simulink model "LR_RL"  (R2021a)
settings: Solver=FixedStepAuto  StartTime=0.0  StopTime=T  FixedStep=Ts  RelTol=1e-3
undefined symbols (not defined in the file): isTerminate, max_theta_error, max_x_error, max_y_error, pLander, references, u0, xpos0
libraries: simulink x8, rllib x1
settings Model: SimulationMode=accelerator  Creator=The MathWorks, Inc.  LastModifiedBy=ldy
settings DataIOCC: ReturnWorkspaceOutputs=off

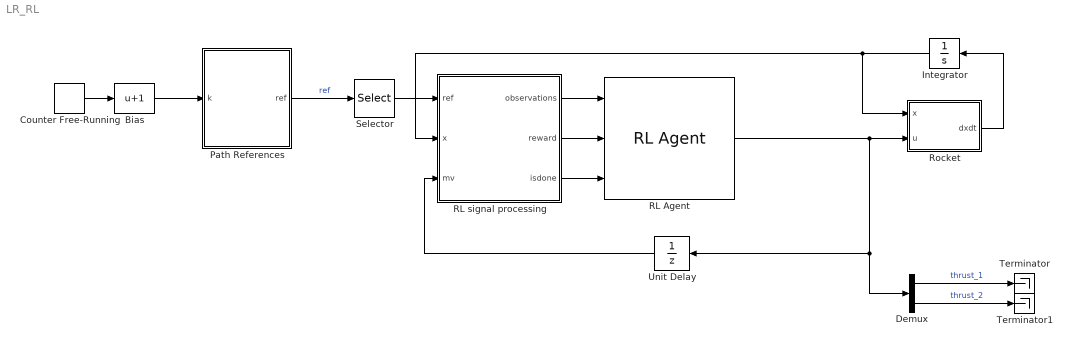
== system LR_RL ==
  Bias : Bias  Bias=1
  Counter Free-Running : simulink/Sources/Counter Free-Running  NumBits=16  tsamp=Ts
  Demux : Demux  Outputs=2
  Integrator : Integrator  InitialCondition=[xpos0;60;0;0;0;0]
  Path References : MATLAB Function  TreatAsAtomicUnit=on
  RL Agent : rllib/RL Agent  Agent=agent  ExternalActionAsInput=off  ProvideCumRwd=off  TreatAsDirectFeedthrough=on
  RL signal processing : Subsystem
  Rocket : MATLAB Function  TreatAsAtomicUnit=on
  Selector : Selector  InputPortWidth=66  IndexOptions=Index vector (dialog)  Indices=[1 2 3 4 5 6]  OutputSizes=1
  Terminator : Terminator
  Terminator1 : Terminator
  Unit Delay : UnitDelay  InitialCondition=u0  SampleTime=-1  HasFrameUpgradeWarning=on
  wires:
  Rocket/1(dxdt) -> Integrator/1
  Integrator/1 -> RL signal processing/2(x), Rocket/1(x)
  Path References/1(ref) -> Selector/1  "ref"
  Counter Free-Running/1 -> Bias/1
  Bias/1 -> Path References/1(k)
  RL signal processing/1(observations) -> RL Agent/1
  RL signal processing/3(isdone) -> RL Agent/3
  RL signal processing/2(reward) -> RL Agent/2
  Selector/1 -> RL signal processing/1(ref)
  Unit Delay/1 -> RL signal processing/3(mv)
  RL Agent/1 -> Unit Delay/1, Demux/1, Rocket/2(u)
  Demux/1 -> Terminator/1  "thrust_1"
  Demux/2 -> Terminator1/1  "thrust_2"

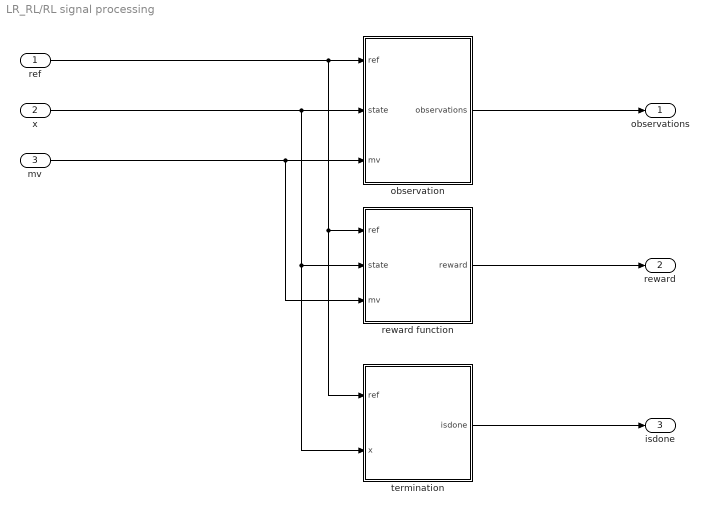
== system LR_RL/RL signal processing ==
  ref : Inport
  x : Inport  Port=2
  mv : Inport  Port=3
  observation : Subsystem
  reward function : Subsystem
  termination : Subsystem
  observations : Outport
  reward : Outport  Port=2
  isdone : Outport  Port=3
  wires:
  observation/1(observations) -> observations/1
  termination/1(isdone) -> isdone/1
  reward function/1(reward) -> reward/1
  ref/1 -> termination/1(ref), reward function/1(ref), observation/1(ref)
  x/1 -> termination/2(x), reward function/2(state), observation/2(state)
  mv/1 -> reward function/3(mv), observation/3(mv)

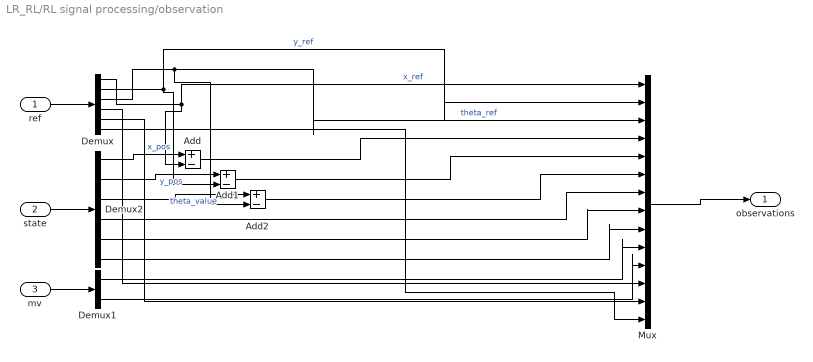
== system LR_RL/RL signal processing/observation ==
  ref : Inport
  state : Inport  Port=2
  mv : Inport  Port=3
  Add : Sum  Inputs=+-
  Add1 : Sum  Inputs=+-
  Add2 : Sum  Inputs=+-
  Demux : Demux  Outputs=6
  Demux1 : Demux  Outputs=2
  Demux2 : Demux  Outputs=6
  Mux : Mux  Inputs=14
  observations : Outport
  wires:
  ref/1 -> Demux/1
  Mux/1 -> observations/1
  mv/1 -> Demux1/1
  state/1 -> Demux2/1
  Demux/1 -> Add/2, Mux/1  "x_ref"
  Demux/2 -> Mux/2, Add1/2  "y_ref"
  Demux/3 -> Add2/2, Mux/3  "theta_ref"
  Demux2/4 -> Mux/7
  Demux2/5 -> Mux/8
  Demux2/6 -> Mux/9
  Demux1/1 -> Mux/10
  Demux1/2 -> Mux/11
  Demux2/1 -> Add/1  "x_pos"
  Add/1 -> Mux/4
  Demux2/2 -> Add1/1  "y_pos"
  Add1/1 -> Mux/5
  Demux2/3 -> Add2/1  "theta_value"
  Add2/1 -> Mux/6
  Demux/4 -> Mux/12
  Demux/5 -> Mux/13
  Demux/6 -> Mux/14

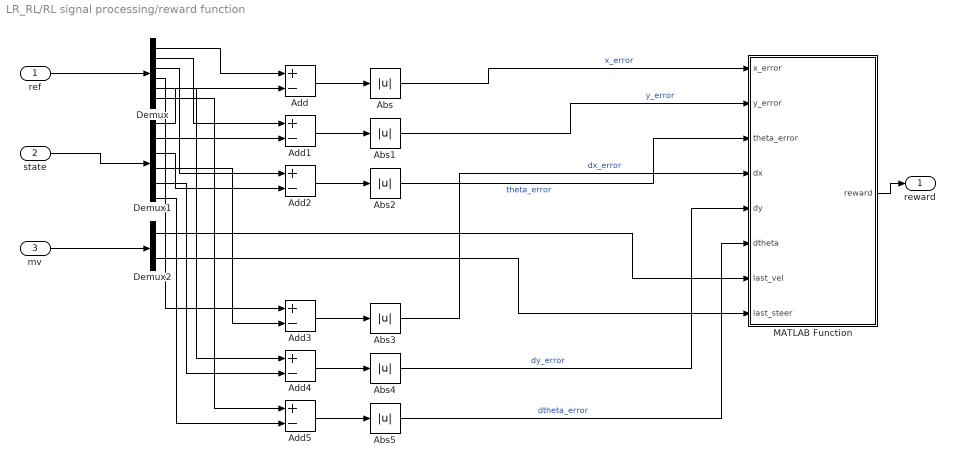
== system LR_RL/RL signal processing/reward function ==
  ref : Inport
  state : Inport  Port=2
  mv : Inport  Port=3
  Abs{,1..5} (6 alike) : Abs
  Add{,1..5} (6 alike) : Sum  Inputs=+-
  Demux : Demux  Outputs=6
  Demux1 : Demux  Outputs=6
  Demux2 : Demux  Outputs=2
  MATLAB Function : MATLAB Function  TreatAsAtomicUnit=on
  reward : Outport
  wires:
  MATLAB Function/1(reward) -> reward/1
  ref/1 -> Demux/1
  state/1 -> Demux1/1
  Demux/1 -> Add/1
  Demux/2 -> Add1/1
  Demux/3 -> Add2/1
  Demux1/1 -> Add/2
  Demux1/2 -> Add1/2
  Demux1/3 -> Add2/2
  Add/1 -> Abs/1
  Add1/1 -> Abs1/1
  Add2/1 -> Abs2/1
  mv/1 -> Demux2/1
  Abs/1 -> MATLAB Function/1(x_error)  "x_error"
  Abs1/1 -> MATLAB Function/2(y_error)  "y_error"
  Abs2/1 -> MATLAB Function/3(theta_error)  "theta_error"
  Demux2/1 -> MATLAB Function/7(last_vel)
  Demux2/2 -> MATLAB Function/8(last_steer)
  Add3/1 -> Abs3/1
  Add4/1 -> Abs4/1
  Add5/1 -> Abs5/1
  Demux/4 -> Add3/1
  Demux1/4 -> Add3/2
  Demux/5 -> Add4/1
  Demux1/5 -> Add4/2
  Demux/6 -> Add5/1
  Demux1/6 -> Add5/2
  Abs3/1 -> MATLAB Function/4(dx)  "dx_error"
  Abs4/1 -> MATLAB Function/5(dy)  "dy_error"
  Abs5/1 -> MATLAB Function/6(dtheta)  "dtheta_error"

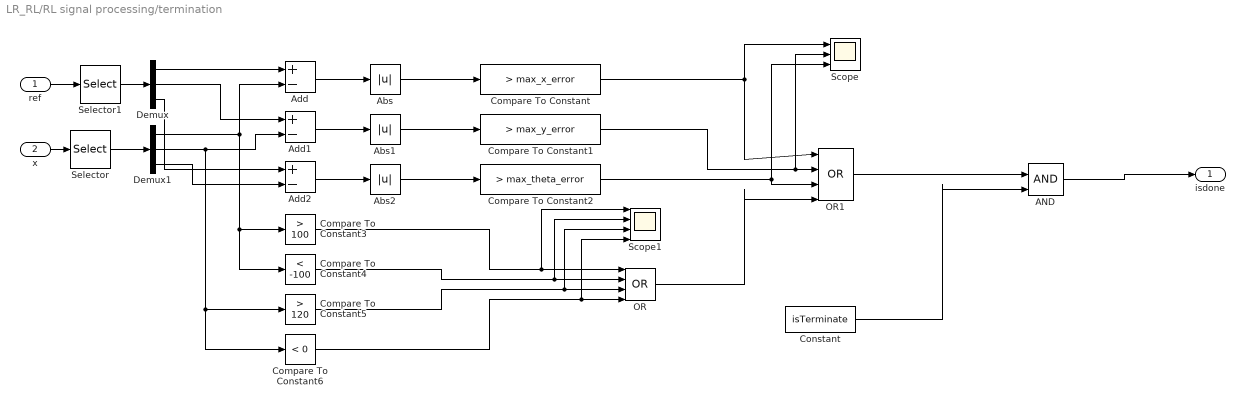
== system LR_RL/RL signal processing/termination ==
  ref : Inport
  x : Inport  Port=2
  AND : Logic  IconShape=distinctive  AllPortsSameDT=off  OutDataTypeStr=boolean
  Abs : Abs
  Abs1 : Abs
  Abs2 : Abs
  Add : Sum  Inputs=+-
  Add1 : Sum  Inputs=+-
  Add2 : Sum  Inputs=+-
  Compare To Constant : simulink/Logic and Bit Operations/Compare To Constant  relop=>  const=max_x_error  OutDataTypeStr=boolean
  Compare To Constant1 : simulink/Logic and Bit Operations/Compare To Constant  relop=>  const=max_y_error  OutDataTypeStr=boolean
  Compare To Constant2 : simulink/Logic and Bit Operations/Compare To Constant  relop=>  const=max_theta_error  OutDataTypeStr=boolean
  Compare To Constant3 : simulink/Logic and Bit Operations/Compare To Constant  relop=>  const=100  OutDataTypeStr=boolean
  Compare To Constant4 : simulink/Logic and Bit Operations/Compare To Constant  relop=<  const=-100  OutDataTypeStr=boolean
  Compare To Constant5 : simulink/Logic and Bit Operations/Compare To Constant  relop=>  const=120  OutDataTypeStr=boolean
  Compare To Constant6 : simulink/Logic and Bit Operations/Compare To Constant  relop=<  const=0  OutDataTypeStr=boolean
  Constant : Constant  Value=isTerminate
  Demux : Demux  Outputs=3
  Demux1 : Demux  Outputs=3
  OR : Logic  Operator=OR  Inputs=4  IconShape=distinctive  AllPortsSameDT=off  OutDataTypeStr=boolean
  OR1 : Logic  Operator=OR  Inputs=4  IconShape=distinctive  AllPortsSameDT=off  OutDataTypeStr=boolean
  Scope : Scope  NumInputPorts=3
  Scope1 : Scope  NumInputPorts=4
  Selector : Selector  InputPortWidth=6  IndexOptions=Index vector (dialog)  Indices=[1 2 3]  OutputSizes=1
  Selector1 : Selector  InputPortWidth=6  IndexOptions=Index vector (dialog)  Indices=[1 2 3]  OutputSizes=1
  isdone : Outport
  wires:
  Add1/1 -> Abs1/1
  Abs/1 -> Compare To Constant/1
  Demux1/2 -> Compare To Constant6/1, Compare To Constant5/1, Add1/2
  Demux1/3 -> Add2/2
  Demux/1 -> Add/1
  Abs2/1 -> Compare To Constant2/1
  Add/1 -> Abs/1
  ref/1 -> Selector1/1
  Demux/3 -> Add2/1
  Selector/1 -> Demux1/1
  Demux/2 -> Add1/1
  Abs1/1 -> Compare To Constant1/1
  x/1 -> Selector/1
  Demux1/1 -> Compare To Constant4/1, Compare To Constant3/1, Add/2
  Add2/1 -> Abs2/1
  Compare To Constant3/1 -> Scope1/1, OR/1
  Compare To Constant4/1 -> Scope1/2, OR/2
  Compare To Constant6/1 -> Scope1/4, OR/4
  Compare To Constant5/1 -> Scope1/3, OR/3
  Compare To Constant/1 -> Scope/1, OR1/1
  Compare To Constant1/1 -> Scope/2, OR1/2
  Compare To Constant2/1 -> OR1/3, Scope/3
  OR/1 -> OR1/4
  Selector1/1 -> Demux/1
  OR1/1 -> AND/1
  AND/1 -> isdone/1
  Constant/1 -> AND/2

== matlab function LR_RL/Path References ==
  data: k input; ref output; references parameter; pLander parameter
function ref = fcn(k,references,pLander)
ref = RocketLanderReferenceSignal(k,references,pLander);

== matlab function LR_RL/Rocket ==
  data: x input; u input; dxdt output
function dxdt = fcn(x,u)
dxdt = RocketStateFcn(x,u);

== matlab function LR_RL/RL signal processing/reward function/MATLAB Function ==
  data: x_error input; reward output; y_error input; theta_error input; dx input; dy input; dtheta input; last_vel input; last_steer input
function reward = reward(x_error, y_error, theta_error,dx, dy,dtheta,last_vel, last_steer)

x_pos = exp(-x_error/3);
y_pos = exp(-y_error/3);
theta_pos = 0.2*exp(-theta_error);

position_pos = x_pos + y_pos + theta_pos;

dx_pos = exp(-dx/3);
dy_pos = exp(-dy/3);
dtheta_pos = exp(-dtheta);
vel_pos = dx_pos + dtheta_pos + dy_pos;

pos_neg = -tanh(x_error/4) -tanh(y_error/5) -tanh(theta_error);

vel_neg = -tanh(dx/5) -tanh(dy/5) -tanh(dtheta);


% reward = position_pos + 0.1*vel_pos + pos_neg + 0.1*vel_neg;
reward = position_pos + 0.1*vel_pos;
% reward = neg_reward;

if x_error < 3
    reward = reward +1;
end

if y_error < 3
    reward = reward +1;
end

if theta_error < 0.5
    reward = reward +0.5;
end

%%
if x_error > 10
    reward = reward -10;
end

if y_error > 10
    reward = reward -10;
end
